simulink model "simpSimuRoboToGoRegelPD"  (R2019b)
settings: Solver=FixedStepDiscrete  StartTime=0.0  StopTime=100  FixedStep=0.1  RelTol=1e-3  EnableMultiTasking=on
libraries: simulink x2, simulink_extras x2, fahrradDiskr x1, cstblocks x1
settings Model: Creator=pic  LastModifiedBy=mackst
settings SolverCC: ZeroCrossAlgorithm=Adaptive  AutoInsertRateTranBlk=on
settings DataIOCC: SaveFormat=Array  TimeSaveName=t  OutputSaveName=y
settings OptimizationCC: ExpressionDepthLimit=2147483647  LifeSpan=inf
settings DebuggingCC: UnderspecifiedInitializationDetection=Classic  MergeDetectMultiDrivingBlocksExec=none  SolverPrmCheckMsg=warning  AllowSymbolicDim=off  StateNameClashWarn=warning  SFUnexpectedBacktrackingDiag=warning  SFNoUnconditionalDefaultTransitionDiag=warning  SFExecutionAtInitializationDiag=none  ArithmeticOperatorsInVariantConditions=warning
settings HardwareCC: ProdBitPerPointer=32  ProdBitPerSizeT=32  ProdBitPerPtrDiffT=32  ProdLargestAtomicFloat=None  ProdIntDivRoundTo=Undefined  ProdEndianess=Unspecified  ProdWordSize=32  ProdHWDeviceType=32-bit Generic
settings ModelReferenceCC: PropagateSignalLabelsOutOfModel=off
settings SFSimCC: SimUseLocalCustomCode=off  CustomCodeUndefinedFunction=UseInterfaceOnly
settings RTWCC: RTWUseLocalCustomCode=off
settings CodeAppCC: StateflowObjectComments=on
settings GRTTargetCC: TargetLangStandard=C89/C90 (ANSI)  CombineOutputUpdateFcns=off  GRTInterface=on
settings ConfigComp: CovMetricSettings=dw  CovSaveCumulativeToWorkspaceVar=on  CovSaveSingleToWorkspaceVar=on  CovExternalEMLEnable=off

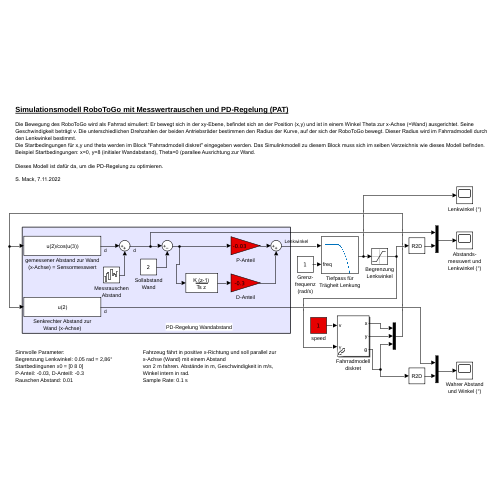
[thumbnail: Simulink's stored preview of the top-level diagram]
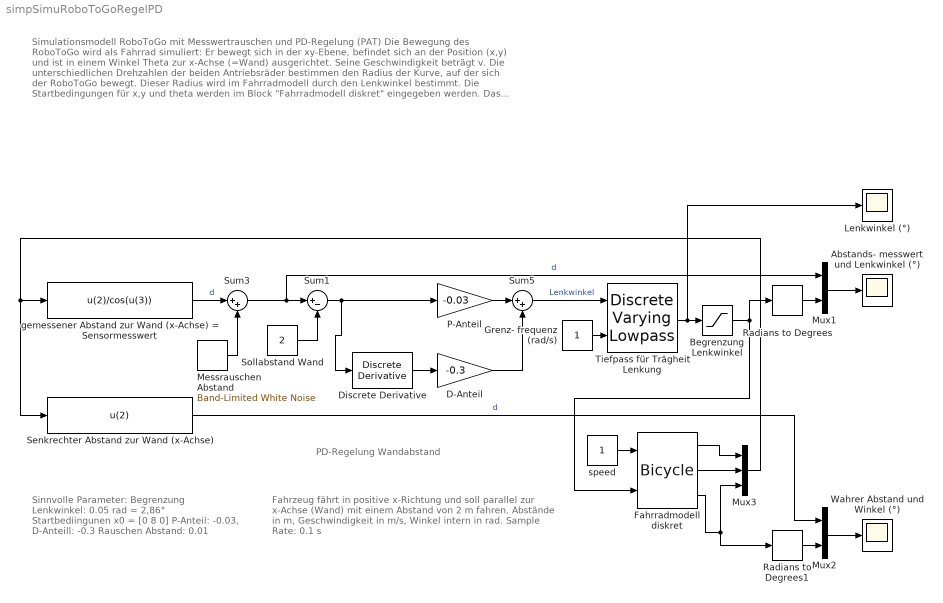
== system simpSimuRoboToGoRegelPD ==
  note: Sinnvolle Parameter:
      | Begrenzung Lenkwinkel: 0.05 rad = 2,86°
      | Startbediingunen x0 = [0 8 0]
      | P-Anteil: -0.03, D-Anteill: -0.3
      | Rauschen Abstand: 0.01
  note: PD-Regelung Wandabstand
  note: Simulationsmodell RoboToGo mit Messwertrauschen und PD-Regelung (PAT)
      |
      | Die Bewegung des RoboToGo wird als Fahrrad simuliert: Er bewegt sich in der xy-Ebene, befindet sich an der Position (x,y) und ist in einem Winkel Theta zur x-Achse (=Wand) ausgerichtet. Seine Geschwindigkeit beträgt v. Die unterschiedlichen Drehzahlen der beiden Antriebsräder bestimmen den Radius der Kurve, auf der sich der RoboToGo bewegt. Dieser Radius wird im Fahrradmodell durch den Lenkwinkel bestimmt.
      | Die Startbedingungen für x,y und theta werden im Block "Fahrradmodell diskret" eingegeben werden. Das Simulinkmodell zu diesem Block muss sich im selben Verzeichnis wie dieses Modell befinden. Beispiel Startbedingungen: x=0, y=8 (initialer Wandabstand), Theta=0 (parallee Ausrichtung zur Wand.
      |
      | Dieses Modell ist dafür da, um die PD-Regelung zu optimieren.
      |
      | S. Mack, 7.11.2022
  note: Fahrzeug fährt in positive x-Richtung und soll parallel zur x-Achse (Wand) mit einem Abstand
      | von 2 m fahren. Abstände in m, Geschwindigkeit in m/s, Winkel intern in rad.
      | Sample Rate: 0.1 s
  Abstands- messwert und Lenkwinkel (°) : Scope
  Begrenzung Lenkwinkel : Saturate  UpperLimit=0.05  LowerLimit=-0.05
  D-Anteil : Gain  Gain=-0.3
  Discrete Derivative : simulink/Discrete/Discrete Derivative  gainval=1.0  ICPrevScaledInput=0.0  OutMin=[]  OutMax=[]  OutDataType=fixdt(1, 16)  OutScaling=2^-10  DoSatur=off
  Fahrradmodell diskret : fahrradDiskr/Vehicles/Bicycle  vlim=1  accel=Inf  alim=Inf  steer_rate=Inf  L=1  x0=[0, 8, 0]
  Grenz- frequenz (rad/s) : Constant  SampleTime=-1
  Lenkwinkel (°) : Scope
  Messrauschen Abstand : simulink/Sources/Band-Limited White Noise  Cov=[0.01]  Ts=0.1  seed=[23341]
  Mux1 : Mux  Inputs=2
  Mux2 : Mux  Inputs=2
  Mux3 : Mux  Inputs=3
  P-Anteil : Gain  Gain=-0.03
  Radians to Degrees : simulink_extras/Transformations/Radians to Degrees
  Radians to Degrees1 : simulink_extras/Transformations/Radians to Degrees
  Senkrechter Abstand zur Wand (x-Achse) : Fcn  Expr=u(2)
  Sollabstand Wand : Constant  Value=2
  Sum1 : Sum  Inputs=|+-
  Sum3 : Sum  Inputs=|++
  Sum5 : Sum  Inputs=|++
  Tiefpass für Trägheit Lenkung : cstblocks/Linear Parameter Varying/Discrete Varying Lowpass  N=2  w0=0  Ts=0.1
      settings: SourceProductBaseCode=CT
  Wahrer Abstand und Winkel (°) : Scope
  gemessener Abstand zur Wand (x-Achse) = Sensormesswert : Fcn  Expr=u(2)/cos(u(3))
  speed : Constant  VectorParams1D=off  SampleTime=-1
  wires:
  Mux3/1 -> Senkrechter Abstand zur Wand (x-Achse)/1, gemessener Abstand zur Wand (x-Achse) = Sensormesswert/1
  speed/1 -> Fahrradmodell diskret/1
  Fahrradmodell diskret/1 -> Mux3/1
  Fahrradmodell diskret/2 -> Mux3/2
  Fahrradmodell diskret/3 -> Radians to Degrees1/1, Mux3/3
  Sum1/1 -> Discrete Derivative/1, P-Anteil/1
  Sollabstand Wand/1 -> Sum1/2
  Sum3/1 -> Mux1/1, Sum1/1  "d"
  Senkrechter Abstand zur Wand (x-Achse)/1 -> Mux2/1  "d"
  Messrauschen Abstand/1 -> Sum3/2
  gemessener Abstand zur Wand (x-Achse) = Sensormesswert/1 -> Sum3/1  "d"
  Mux2/1 -> Wahrer Abstand und Winkel (°)/1
  Mux1/1 -> Abstands- messwert und Lenkwinkel (°)/1
  Radians to Degrees/1 -> Mux1/2
  Radians to Degrees1/1 -> Mux2/2
  Grenz- frequenz (rad/s)/1 -> Tiefpass für Trägheit Lenkung/2
  Begrenzung Lenkwinkel/1 -> Radians to Degrees/1, Fahrradmodell diskret/2
  Sum5/1 -> Tiefpass für Trägheit Lenkung/1  "Lenkwinkel"
  P-Anteil/1 -> Sum5/1
  D-Anteil/1 -> Sum5/2
  Discrete Derivative/1 -> D-Anteil/1
  Tiefpass für Trägheit Lenkung/1 -> Lenkwinkel (°)/1, Begrenzung Lenkwinkel/1
